simulink model "PI_boucle_ouverte"  (R2024a)
settings: Solver=VariableStepAuto  StartTime=0.0  StopTime=10.0  RelTol=1e-3
undefined symbols (not defined in the file): A, B, C, D, x0
settings Model: Creator=DELL  LastModifiedBy=DELL

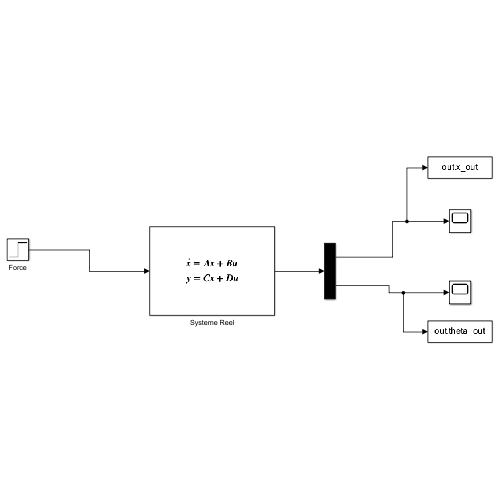
[thumbnail: Simulink's stored preview of the top-level diagram]
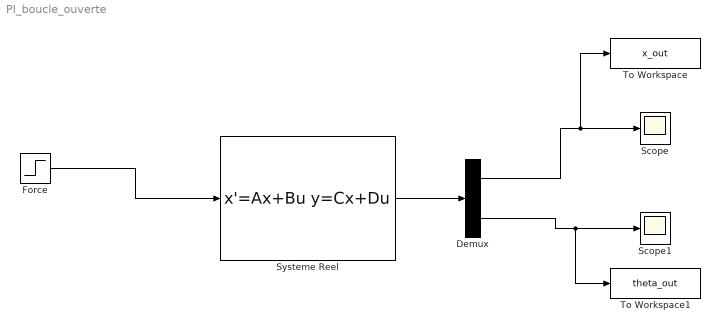
== system PI_boucle_ouverte ==
  Demux : Demux  Outputs=2
  Force : Step  Time=0.5  SampleTime=0
  Scope : Scope
  Scope1 : Scope
  Systeme Reel : StateSpace  A=A  B=B  C=C  D=D  InitialCondition=x0
  To Workspace : ToWorkspace  VariableName=x_out  SaveFormat=Timeseries  SampleTime=-1
  To Workspace1 : ToWorkspace  VariableName=theta_out  SaveFormat=Timeseries  SampleTime=-1
  wires:
  Systeme Reel/1 -> Demux/1
  Demux/1 -> To Workspace/1, Scope/1
  Demux/2 -> To Workspace1/1, Scope1/1
  Force/1 -> Systeme Reel/1
